simulink model "x2_myfoc_transform"  (R2025b)
settings: Solver=ode23t  StartTime=0.0  StopTime=0.5  RelTol=1e-3
values from neighbouring files (symbols this model uses):
  my_Ts = 1/SwitchFrequency    (= 5e-05)    [foc_para.m]
  Tpwm = 4000-1    (= 3999)    [foc_para.m]
  vbus = 12    [foc_para.m]
undefined symbols (not defined in the file or in its folder): DiscIntNeverNeededParam
settings Model: Creator=disnox  LastModifiedBy=yolo
settings DataIOCC: ReturnWorkspaceOutputs=off
settings DebuggingCC: SaveWithParameterizedLinksMsg=none  ParameterPrecisionLossMsg=none
settings HardwareCC: ProdBitPerPointer=32.0  ProdBitPerSizeT=32.0  ProdBitPerPtrDiffT=32.0  ProdLargestAtomicInteger=Long  ProdLargestAtomicFloat=Double  ProdWordSize=32.0  ProdHWDeviceType=ARM Compatible->ARM Cortex-M
settings RTWCC: GPUComputeCapability=3.5

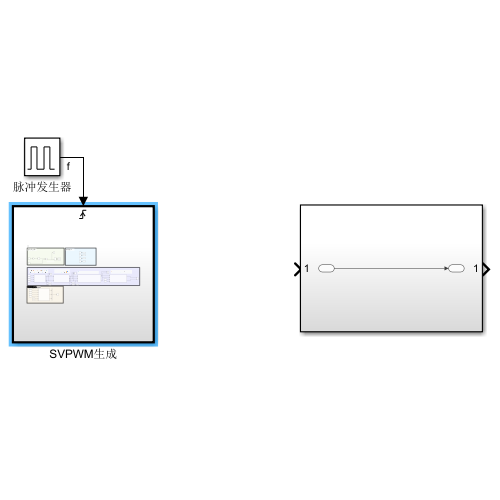
[thumbnail: Simulink's stored preview of the top-level diagram]
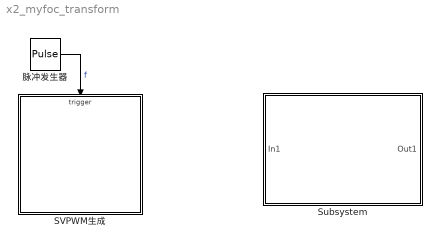
== system x2_myfoc_transform ==
  SVPWM生成 : Subsystem
  Subsystem : Subsystem
  脉冲发生器 : DiscretePulseGenerator  PulseType=Time based  Period=my_Ts  PulseWidth=5
  wires:
  脉冲发生器/1 -> SVPWM生成/Trigger  "f"

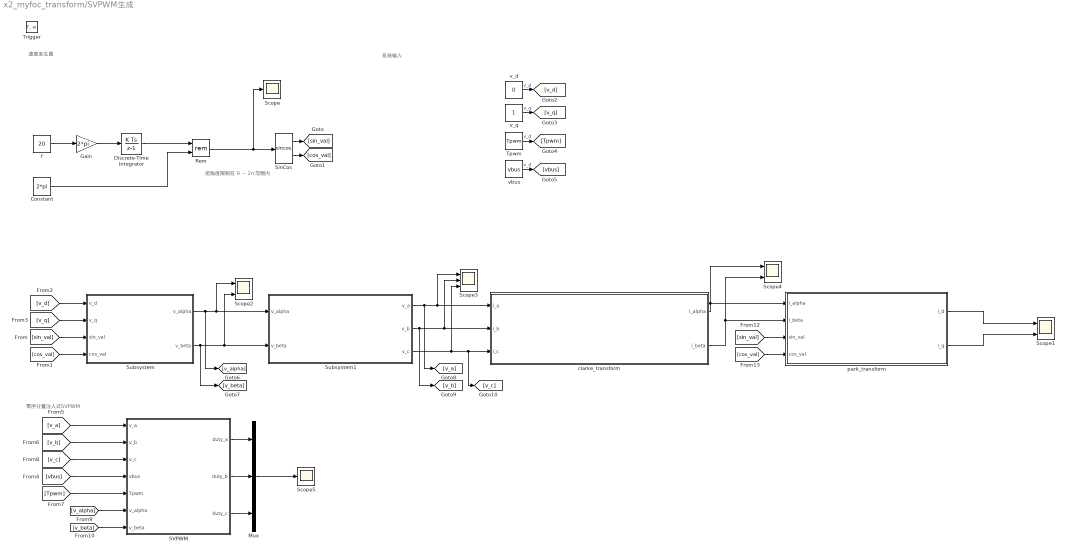
== system x2_myfoc_transform/SVPWM生成 ==
  note: 零序分量注入式SVPWM
  note: 系统输入
  note: 把角度限制在 0 ~ 2π 范围内
  note: 速度发生器
  Trigger : TriggerPort  VariantControl=(inherit)  PortDimensions=1
  Constant : Constant  Value=2*pi
  Discrete-Time Integrator : DiscreteIntegrator  SampleTime=-1  ICPrevOutput=DiscIntNeverNeededParam  ICPrevScaledInput=DiscIntNeverNeededParam
  Gain : Gain  Gain=2*pi
  Mux : Mux  Inputs=3
  Rem : Math  Operator=rem
  SVPWM : Subsystem
  Scope : Scope
      settings: ActiveDisplayYMinimum=4.21833  ActiveDisplayYMaximum=5.47784  DataLoggingVariableName=ScopeData4
  Scope1 : Scope  NumInputPorts=2
      settings: ActiveDisplayYMinimum=-0.125  ActiveDisplayYMaximum=1.125  DataLoggingVariableName=ScopeData6
  Scope2 : Scope  NumInputPorts=2
      settings: ActiveDisplayYMinimum=-0.125  ActiveDisplayYMaximum=1.125
  Scope3 : Scope  NumInputPorts=3
      settings: ActiveDisplayYMinimum=0.45152726353160721  ActiveDisplayYMaximum=0.8626163459637548
  Scope4 : Scope  NumInputPorts=2
      settings: ActiveDisplayYMinimum=-0.125  ActiveDisplayYMaximum=1.125  DataLoggingVariableName=ScopeData2
  Scope5 : Scope
      settings: ActiveDisplayYMinimum=1516.2285901685057  ActiveDisplayYMaximum=2483.1175310559743  DataLoggingVariableName=ScopeData10
  SinCos : Trigonometry  Operator=sincos
  Subsystem : Subsystem
  Subsystem1 : Subsystem
  Tpwm : Constant  Value=Tpwm
  clarke_transform : Subsystem  TreatAsAtomicUnit=on
      settings: RTWSystemCode=Nonreusable function  RTWFcnNameOpts=Use subsystem name
  f : Constant  Value=20
  park_transform : Subsystem  TreatAsAtomicUnit=on
      settings: RTWSystemCode=Nonreusable function  RTWFcnNameOpts=Use subsystem name
  v_d : Constant  Value=0
  v_q : Constant
  vbus : Constant  Value=vbus
  wires:
  SinCos/2 -> [cos_val]
  Constant/1 -> Rem/2
  Gain/1 -> Discrete-Time Integrator/1
  f/1 -> Gain/1
  SinCos/1 -> [sin_val]
  Discrete-Time Integrator/1 -> Rem/1
  Rem/1 -> SinCos/1, Scope/1
  v_d/1 -> [v_d]  "v_d"
  v_q/1 -> [v_q]  "v_q"
  [v_d] -> Subsystem/1(v_d)
  [v_q] -> Subsystem/2(v_q)
  [sin_val] -> Subsystem/3(sin_val)
  [cos_val] -> Subsystem/4(cos_val)
  Subsystem/1(v_alpha) -> [v_alpha], Scope2/1, Subsystem1/1(v_alpha)
  Subsystem/2(v_beta) -> [v_beta], Scope2/2, Subsystem1/2(v_beta)
  Subsystem1/1(v_a) -> [v_a], Scope3/1, clarke_transform/1(i_a)
  Subsystem1/2(v_b) -> [v_b], Scope3/2, clarke_transform/2(i_b)
  Subsystem1/3(v_c) -> Scope3/3, [v_c], clarke_transform/3(i_c)
  park_transform/1(i_d) -> Scope1/1
  [cos_val] -> park_transform/4(cos_val)
  park_transform/2(i_q) -> Scope1/2
  [sin_val] -> park_transform/3(sin_val)
  clarke_transform/1(i_alpha) -> Scope4/1, park_transform/1(i_alpha)
  clarke_transform/2(i_beta) -> Scope4/2, park_transform/2(i_beta)
  Tpwm/1 -> [Tpwm]  "v_d"
  vbus/1 -> [vbus]  "v_d"
  [v_a] -> SVPWM/1(v_a)
  [v_b] -> SVPWM/2(v_b)
  [v_c] -> SVPWM/3(v_c)
  [vbus] -> SVPWM/4(vbus)
  [Tpwm] -> SVPWM/5(Tpwm)
  [v_alpha] -> SVPWM/6(v_alpha)
  [v_beta] -> SVPWM/7(v_beta)
  SVPWM/1(duty_a) -> Mux/1
  SVPWM/2(duty_b) -> Mux/2
  SVPWM/3(duty_c) -> Mux/3
  Mux/1 -> Scope5/1

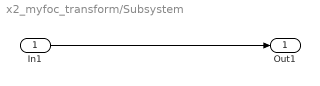
== system x2_myfoc_transform/Subsystem ==
  In1 : Inport
  Out1 : Outport
  wires:
  In1/1 -> Out1/1

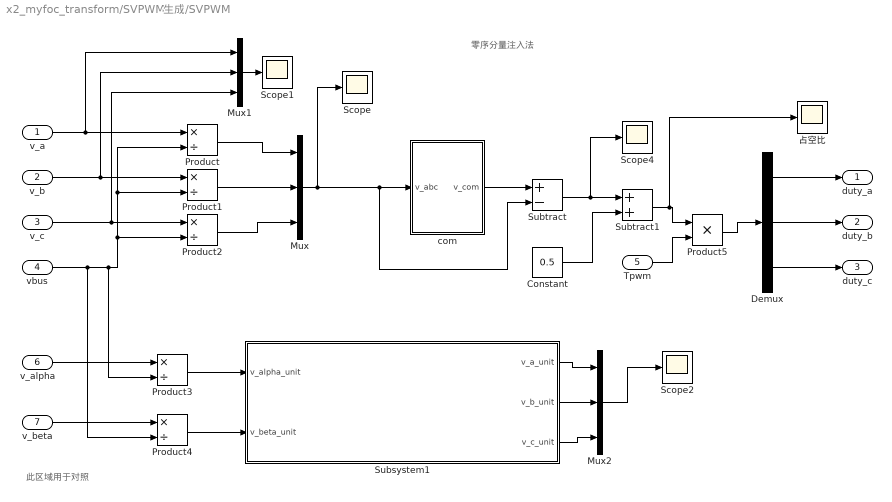
== system x2_myfoc_transform/SVPWM生成/SVPWM ==
  note: 零序分量注入法
  note: 此区域用于对照
  v_a : Inport
  v_b : Inport  Port=2
  v_c : Inport  Port=3
  vbus : Inport  Port=4
  Tpwm : Inport  Port=5
  v_alpha : Inport  Port=6
  v_beta : Inport  Port=7
  Constant : Constant  Value=0.5
  Demux : Demux  Outputs=3
  Mux : Mux  Inputs=3
  Mux1 : Mux  Inputs=3
  Mux2 : Mux  Inputs=3
  Product{,1..4} (5 alike) : Product  Inputs=*/
  Product5 : Product
  Scope{,1..2,4} (4 alike) : Scope
      Scope settings: ActiveDisplayYMinimum=-0.037119980202717284  ActiveDisplayYMaximum=0.12611463781154517  DataLoggingVariableName=ScopeData3
      Scope1 settings: ActiveDisplayYMinimum=-1.25  ActiveDisplayYMaximum=1.25  DataLoggingVariableName=ScopeData5
      Scope2 settings: ActiveDisplayYMinimum=-0.10961429555823364  ActiveDisplayYMaximum=0.1562776966292666  DataLoggingVariableName=ScopeData7
      Scope4 settings: ActiveDisplayYMinimum=-0.10096338896491379  ActiveDisplayYMaximum=0.097951820966824463  DataLoggingVariableName=ScopeData9
  Subsystem1 : Subsystem
  Subtract : Sum  Inputs=+-
  Subtract1 : Sum
  com : Subsystem
  占空比 : Scope
      settings: ActiveDisplayYMinimum=0.40978902043912097  ActiveDisplayYMaximum=0.59021097956087909  DataLoggingVariableName=ScopeData8
  duty_a : Outport
  duty_b : Outport  Port=2
  duty_c : Outport  Port=3
  wires:
  v_a/1 -> Mux1/1, Product/1
  vbus/1 -> Product4/2, Product3/2, Product1/2, Product/2, Product2/2
  v_b/1 -> Mux1/2, Product1/1
  v_c/1 -> Mux1/3, Product2/1
  Product/1 -> Mux/1
  Product1/1 -> Mux/2
  Product2/1 -> Mux/3
  Mux/1 -> Subtract/2, com/1(v_abc), Scope/1
  Mux1/1 -> Scope1/1
  v_alpha/1 -> Product3/1
  v_beta/1 -> Product4/1
  Product3/1 -> Subsystem1/1(v_alpha_unit)
  Product4/1 -> Subsystem1/2(v_beta_unit)
  Subsystem1/1(v_a_unit) -> Mux2/1
  Subsystem1/2(v_b_unit) -> Mux2/2
  Subsystem1/3(v_c_unit) -> Mux2/3
  Mux2/1 -> Scope2/1
  com/1(v_com) -> Subtract/1
  Subtract/1 -> Scope4/1, Subtract1/1
  Constant/1 -> Subtract1/2
  Subtract1/1 -> 占空比/1, Product5/1
  Tpwm/1 -> Product5/2
  Product5/1 -> Demux/1
  Demux/1 -> duty_a/1
  Demux/2 -> duty_b/1
  Demux/3 -> duty_c/1

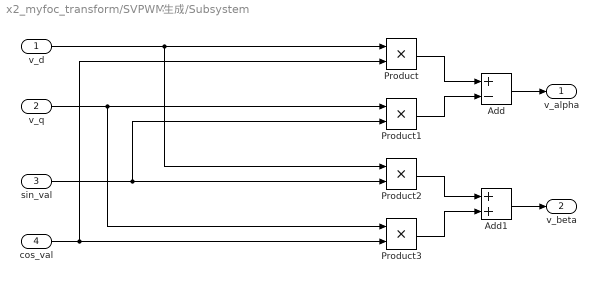
== system x2_myfoc_transform/SVPWM生成/Subsystem ==
  v_d : Inport
  v_q : Inport  Port=2
  sin_val : Inport  Port=3
  cos_val : Inport  Port=4
  Add : Sum  Inputs=+-
  Add1 : Sum  AccumDataTypeStr=double
  Product{,1..3} (4 alike) : Product
  v_alpha : Outport
  v_beta : Outport  Port=2
  wires:
  Add1/1 -> v_beta/1
  v_q/1 -> Product1/1, Product3/1
  Add/1 -> v_alpha/1
  Product/1 -> Add/1
  Product1/1 -> Add/2
  Product2/1 -> Add1/1
  sin_val/1 -> Product2/2, Product1/2
  v_d/1 -> Product2/1, Product/1
  Product3/1 -> Add1/2
  cos_val/1 -> Product3/2, Product/2

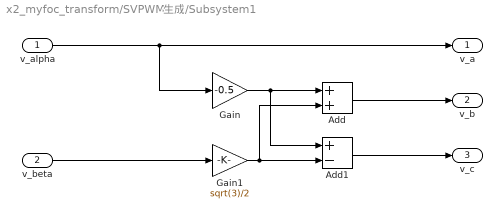
== system x2_myfoc_transform/SVPWM生成/Subsystem1 ==
  v_alpha : Inport
  v_beta : Inport  Port=2
  Add : Sum
  Add1 : Sum  Inputs=+-
  Gain : Gain  Gain=-0.5
  Gain1 : Gain  Gain=sqrt(3)/2
  v_a : Outport
  v_b : Outport  Port=2
  v_c : Outport  Port=3
  wires:
  Gain/1 -> Add1/1, Add/1
  Add1/1 -> v_c/1
  Add/1 -> v_b/1
  Gain1/1 -> Add/2, Add1/2
  v_alpha/1 -> Gain/1, v_a/1
  v_beta/1 -> Gain1/1

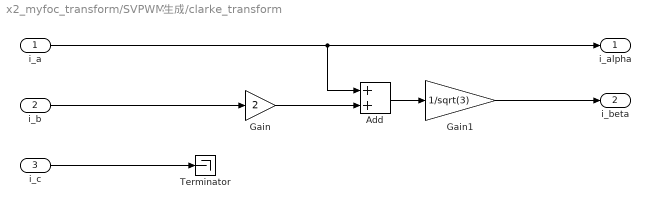
== system x2_myfoc_transform/SVPWM生成/clarke_transform ==
  i_a : Inport
  i_b : Inport  Port=2
  i_c : Inport  Port=3
  Add : Sum
  Gain : Gain  Gain=2
  Gain1 : Gain  Gain=1/sqrt(3)
  Terminator : Terminator
  i_alpha : Outport
  i_beta : Outport  Port=2
  wires:
  i_a/1 -> Add/1, i_alpha/1
  i_b/1 -> Gain/1
  Gain/1 -> Add/2
  Add/1 -> Gain1/1
  Gain1/1 -> i_beta/1
  i_c/1 -> Terminator/1

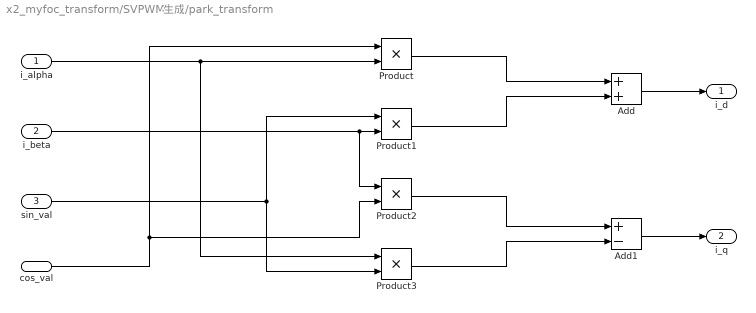
== system x2_myfoc_transform/SVPWM生成/park_transform ==
  i_alpha : Inport
  i_beta : Inport  Port=2
  sin_val : Inport  Port=3
  cos_val : Inport  Port=4
  Add : Sum
  Add1 : Sum  Inputs=+-
  Product{,1..3} (4 alike) : Product
  i_d : Outport
  i_q : Outport  Port=2
  wires:
  i_alpha/1 -> Product/2, Product3/1
  cos_val/1 -> Product2/2, Product/1
  sin_val/1 -> Product3/2, Product1/1
  i_beta/1 -> Product2/1, Product1/2
  Product/1 -> Add/1
  Product1/1 -> Add/2
  Add/1 -> i_d/1
  Product2/1 -> Add1/1
  Product3/1 -> Add1/2
  Add1/1 -> i_q/1

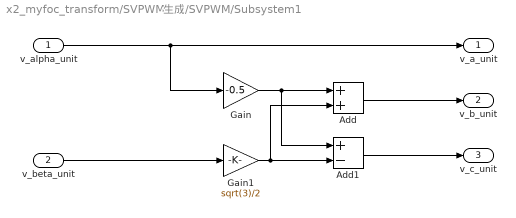
== system x2_myfoc_transform/SVPWM生成/SVPWM/Subsystem1 ==
  v_alpha_unit : Inport
  v_beta_unit : Inport  Port=2
  Add : Sum
  Add1 : Sum  Inputs=+-
  Gain : Gain  Gain=-0.5
  Gain1 : Gain  Gain=sqrt(3)/2
  v_a_unit : Outport
  v_b_unit : Outport  Port=2
  v_c_unit : Outport  Port=3
  wires:
  Gain/1 -> Add1/1, Add/1
  Add1/1 -> v_c_unit/1
  Add/1 -> v_b_unit/1
  Gain1/1 -> Add/2, Add1/2
  v_alpha_unit/1 -> Gain/1, v_a_unit/1
  v_beta_unit/1 -> Gain1/1

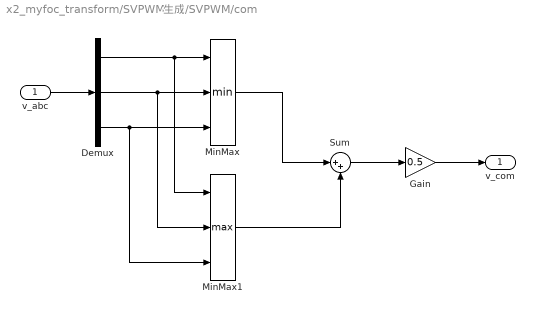
== system x2_myfoc_transform/SVPWM生成/SVPWM/com ==
  v_abc : Inport
  Demux : Demux  Outputs=3
  Gain : Gain  Gain=0.5
  MinMax : MinMax  Inputs=3
  MinMax1 : MinMax  Function=max  Inputs=3
  Sum : Sum  Inputs=|++
  v_com : Outport
  wires:
  v_abc/1 -> Demux/1
  Demux/1 -> MinMax1/1, MinMax/1
  Demux/2 -> MinMax1/2, MinMax/2
  Demux/3 -> MinMax1/3, MinMax/3
  MinMax/1 -> Sum/1
  MinMax1/1 -> Sum/2
  Sum/1 -> Gain/1
  Gain/1 -> v_com/1
